simulink model "mpc"  (R2019b)
settings: Solver=FixedStepAuto  StartTime=0.0  StopTime=100.0  FixedStep=1  RelTol=1e-3
values from neighbouring files (symbols this model uses):
  ausgangsVektor_cT = [0 , 1]    [init.m]    (also in matlab.mat = [1 1])
  durchgriffsVektor_d = [l , -lh/v]    [init.m]    (also in matlab.mat = [0.25 -0.0625])
  eingangsMatrix_B = [0 , 0 ; v, -1]    [init.m]    (also in matlab.mat = [0  0; 2  -1])
  regelMatrix_K = [b a ; b a]    [init.m]    (also in matlab.mat = [50  20; 50  20])
  systemMatrix_A = [0 , v ; 0 , 0]    [init.m]    (also in matlab.mat = [0  2; 0  0])
libraries: mpclib x1

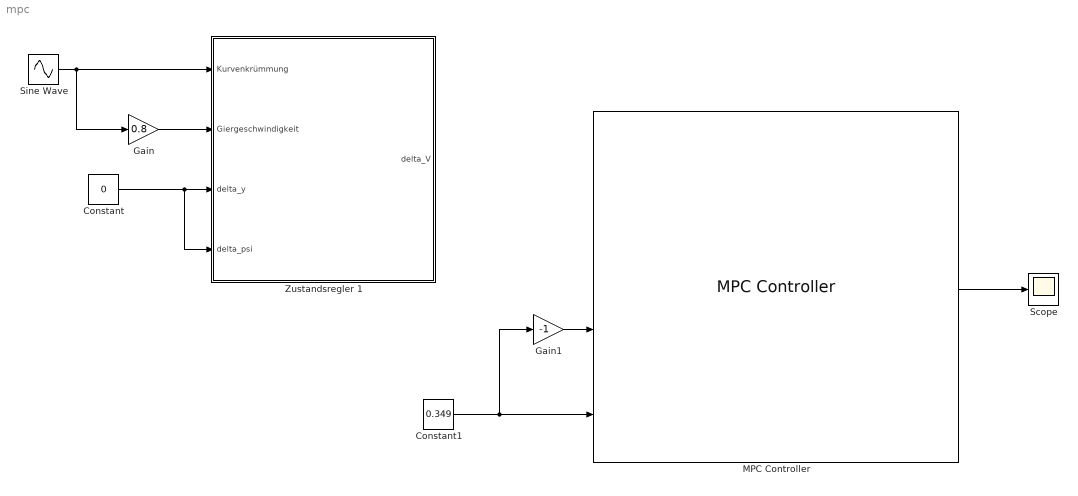
== system mpc ==
  Constant : Constant  Value=0
  Constant1 : Constant  Value=0.349
  Gain : Gain  Gain=0.8
  Gain1 : Gain  Gain=-1
  MPC Controller : mpclib/MPC Controller  SCDEnableBlockLinearizationSpecification=on  is_multiple=0  enable_value=0  return_u0=off  updateMPCinCallerWorkspace=on  md_inport=off  mv_inport=off  uref_inport=off  return_cost=off  return_mvseq=off  return_qpstatus=off  return_xseq=off  return_state=off  return_ovseq=off  state_inport=off  umin_inport=off  umax_inport=off  ymin_inport=on  ymax_inport=on  cc_inport=off  ywt_inport=off  uwt_inport=off  duwt_inport=off  rhoeps_inport=off  pm_inport=off  MaximumP=10  HorizonChoice=FixedHorizon  n_ts=1  n_p=10  n_mv=1  n_md=1  n_ud=0  n_mo=1  n_uo=0  BlockDataType=double  SampleTimeInherited=off  switch_inport=off
  Scope : Scope
  Sine Wave : Sin  SampleTime=0
  Zustandsregler 1 : Subsystem
  wires:
  Constant/1 -> Zustandsregler 1/3(delta_y), Zustandsregler 1/4(delta_psi)
  Sine Wave/1 -> Zustandsregler 1/1("Kurvenkrümmung "), Gain/1
  MPC Controller/1 -> Scope/1
  Gain/1 -> Zustandsregler 1/2("Giergeschwindigkeit ")
  Constant1/1 -> MPC Controller/4, Gain1/1
  Gain1/1 -> MPC Controller/3

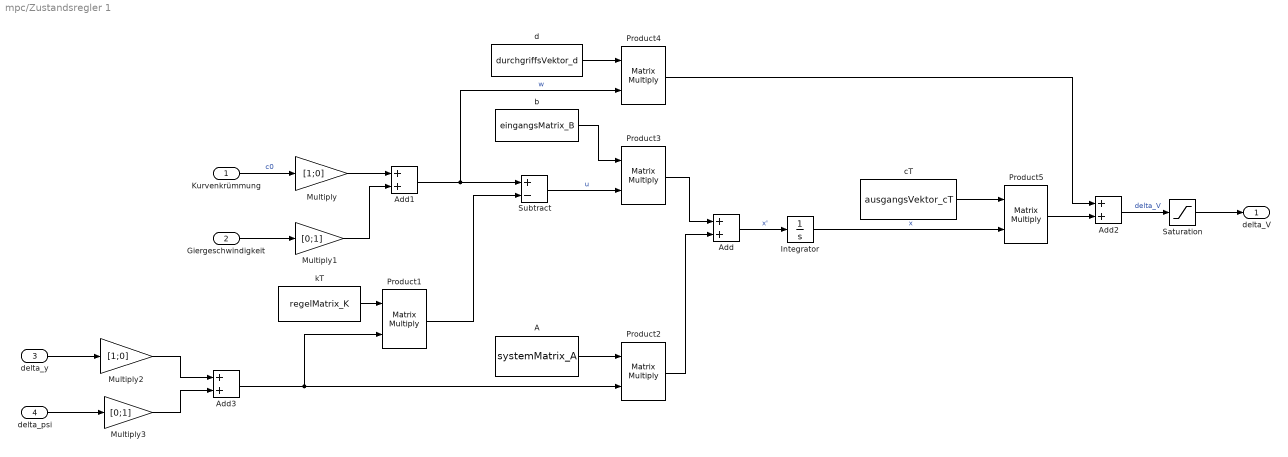
== system mpc/Zustandsregler 1 ==
  "Kurvenkrümmung " : Inport
  "Giergeschwindigkeit " : Inport  Port=2
  delta_y : Inport  Port=3
  delta_psi : Inport  Port=4
  A : Constant  Value=systemMatrix_A  VectorParams1D=off
  Add{,1..3} (4 alike) : Sum
  Integrator : Integrator
  Multiply : Gain  Gain=[1;0]
  Multiply1 : Gain  Gain=[0;1]
  Multiply2 : Gain  Gain=[1;0]
  Multiply3 : Gain  Gain=[0;1]
  Product{1..5} (5 alike) : Product  Multiplication=Matrix(*)
  Saturation : Saturate  UpperLimit=0.349  LowerLimit=-0.349
  Subtract : Sum  Inputs=+-
  b : Constant  Value=eingangsMatrix_B  VectorParams1D=off
  cT : Constant  Value=ausgangsVektor_cT  VectorParams1D=off
  d : Constant  Value=durchgriffsVektor_d  VectorParams1D=off
  kT : Constant  Value=regelMatrix_K  VectorParams1D=off
  delta_V : Outport
  wires:
  Product1/1 -> Subtract/2
  cT/1 -> Product5/1
  Integrator/1 -> Product5/2  "x"
  Add/1 -> Integrator/1  "x'"
  "Kurvenkrümmung "/1 -> Multiply/1  "c0"
  A/1 -> Product2/1
  Product3/1 -> Add/1
  kT/1 -> Product1/1
  Add2/1 -> Saturation/1  "delta_V"
  b/1 -> Product3/1
  Subtract/1 -> Product3/2  "u"
  Multiply/1 -> Add1/1
  Add1/1 -> Product4/2, Subtract/1  "w"
  Multiply1/1 -> Add1/2
  Product2/1 -> Add/2
  "Giergeschwindigkeit "/1 -> Multiply1/1
  delta_y/1 -> Multiply2/1
  Saturation/1 -> delta_V/1
  d/1 -> Product4/1
  Product5/1 -> Add2/2
  Multiply2/1 -> Add3/1
  Multiply3/1 -> Add3/2
  Add3/1 -> Product1/2, Product2/2
  delta_psi/1 -> Multiply3/1
  Product4/1 -> Add2/1
